simulink model "R_Mode_beta6"  (R2020a)
settings: Solver=FixedStepAuto  StartTime=0.0  StopTime=10.0  FixedStep=1e-3  RelTol=1e-3  EnableMultiTasking=on
undefined symbols (not defined in the file): D0, D1, D10, D11, D12, D13, D2, D3, D4, D5, D6, D7, D8, D9, PTA0, PTA1, PTA2, PTB23, PTB9, PTC16, PTC17, PTC2, PTC3, PTC4, PTD0, PTD1, PTD2, PTD3, square
libraries: frdmk64flib x20, simulink x2
settings Model: ExtModeTrigDuration=5  Creator=forre  LastModifiedBy=forre
settings OptimizationCC: EnhancedBackFolding=on  PassReuseOutputArgsAs=Individual arguments  ZeroExternalMemoryAtStartup=off  ZeroInternalMemoryAtStartup=off  MaxStackSize=64  OptimizeBlockOrder=speed  DifferentSizesBufferReuse=on  OptimizationCustomize=off  EfficientTunableParamExpr=on
settings DebuggingCC: ParameterTunabilityLossMsg=error
settings HardwareCC: ProdBitPerPointer=32  ProdBitPerSizeT=32  ProdBitPerPtrDiffT=32  ProdLargestAtomicInteger=Long  ProdLargestAtomicFloat=Double  ProdWordSize=32  ProdHWDeviceType=ARM Compatible->ARM Cortex
settings SFSimCC: MATLABDynamicMemAlloc=off
settings RTWCC: SystemTargetFile=ert.tlc  HardwareBoard=NXP FRDM-K64F  TemplateMakefile=ert_default_tmf  Toolchain=GNU Tools for ARM Embedded Processors
settings CodeAppCC: ForceParamTrailComments=on  IgnoreCustomStorageClasses=off  OperatorAnnotations=on  SimulinkDataObjDesc=on  SFDataObjDesc=on  InsertBlockDesc=on

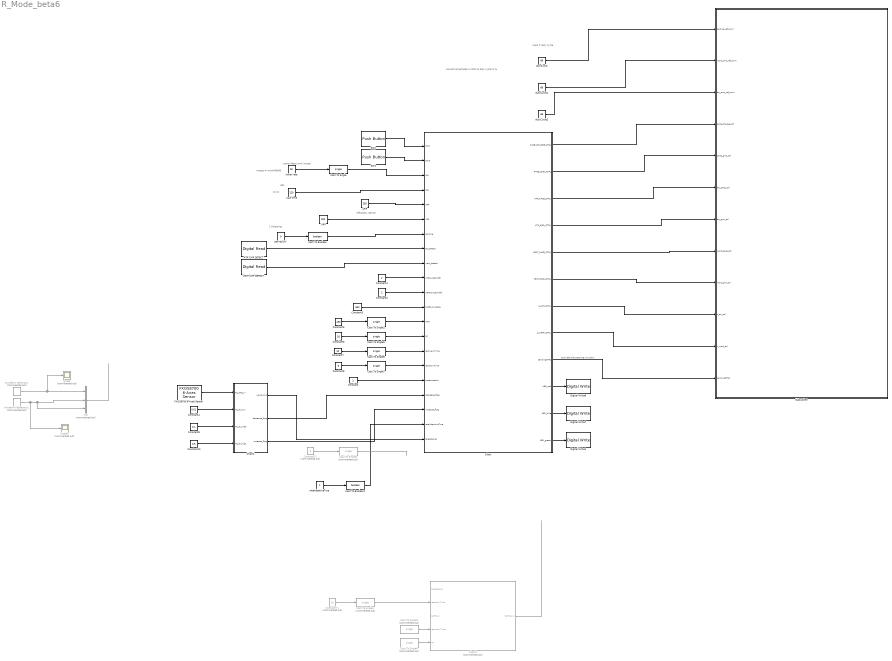
== system R_Mode_beta6 ==
  note: convert amplitude in Volts to duty cycle in %
  note: *****
  note: msecs = mins*60000
  note: URL
  note: refractory period
  note: Lower Rate Limit (msec)
  note: activate the sensing circuitry.
  note: input = duty cycle
  note: 1 if sensing
  ARP : Constant  Value=250
  ATR CMP DETECT : frdmk64flib/Digital Read  Whichpin=PTC16 (D0)  SampleTime=-1
  Cast To Boolean : DataTypeConversion  OutDataTypeStr=boolean
  Cast To Boolean1 : DataTypeConversion  OutDataTypeStr=boolean
  Cast To Single{,1,5..7} (5 alike) : DataTypeConversion  OutDataTypeStr=single
  Cast To Single{2..4,8} (4 alike) : DataTypeConversion  Commented=on  OutDataTypeStr=single
  Chart : Stateflow chart  TreatAsAtomicUnit=on
  Chart1 : Stateflow chart  TreatAsAtomicUnit=on
      settings: PortSchema="{\"entries\":[{\"content\":{\"sides\":[{\"content\":{\"connectorIds\":[\"In1\",\"In2\",\"In3\",\"In4\"]},\"type\":\"ConnectorPlacement.EquallySpacedRectSide\",\"uuid\":\"1efe160a-bf9a-41df-b710-bd83ffcce0b4\"},{\"content\":{\"connectorIds\":[\"Out1\",\"Out3\",\"Out2\"],\"side\":\"RIGHT\"},\"type\":\"ConnectorPlacement.EquallySpacedRectSide\",\"uuid\":\"ac30f416-04bb-4c91-9400-e1e71b20eb48\"},{\"content\":{\"connectorIds\":[],\"side\":\"TOP\"},\"type\":\"ConnectorPlacement.EquallySpacedRectSide\",\"uuid\":\"2c13bf7e-a139-4786-92e7-3ebc0a2be541\"}]},\"type\":\"ConnectorPlacement.EquallySpacedConnector\",\"uuid\":\"36ae9f3c-1d99-4fa5-b372-be33db95aa7c\"}],\"packageUris\":[\"http://schema.mathworks.com/mf0/Connector/19700101\"],\"version\":\"1.0\"}"
  Chart2 : Stateflow chart  Commented=on  TreatAsAtomicUnit=on
  Constant : Constant  Value=2  OutDataTypeStr=double
  Constant1 : Constant  Value=2
  Constant10 : Constant  Value=0.5  OutDataTypeStr=double
  Constant11 : Constant  Commented=on  Value=10  OutDataTypeStr=double
  Constant12 : Constant  Commented=on  Value=3  OutDataTypeStr=double
  Constant2 : Constant  Value=2
  Constant3 : Constant  Value=500
  Constant4 : Constant  Value=0.01  OutDataTypeStr=double
  Constant5 : Constant  Value=150  OutDataTypeStr=double
  Constant6 : Constant  Value=16  OutDataTypeStr=double
  Constant7 : Constant  Value=10  OutDataTypeStr=double
  Constant8 : Constant  Value=5  OutDataTypeStr=double
  Constant9 : Constant  Value=0.1  OutDataTypeStr=double
  Digital Write1 : frdmk64flib/Digital Write  Whichpin=GREEN_LED
  Digital Write6 : frdmk64flib/Digital Write  Whichpin=RED_LED
  Digital Write7 : frdmk64flib/Digital Write  Whichpin=BLUE_LED
  FXOS8700 6-Axes Sensor : frdmk64flib/FXOS8700 6-Axes Sensor  Activesensor=Accelerometer only  ODR=800Hz  HybridODR=400Hz  Accelfullrange=-2g to +2g  SampleTime=-1
  Mux : Mux  Commented=on  Inputs=3
  SW2 : frdmk64flib/Push Button  Whichswitch=SW2  SampleTime1=-1
  SW3 : frdmk64flib/Push Button  Whichswitch=SW3  SampleTime1=-1
  Scope : Scope  Commented=on
  Scope1 : Scope  Commented=on
  Subsystem : Subsystem
  VENT CMP DETECT : frdmk64flib/Digital Read  Whichpin=PTC17 (D1)  SampleTime=-1
  VRP : Constant  Value=250
  Waveform Generator : simulink/Sources/Waveform Generator  Commented=on  OutMin=[]  OutMax=[]  OutDataTypeStr=double  SelectedSignal=1  Signals=square(1,5,10,0)  BlockNames=MultiportSwitch_f97ce9ea1487498  SampleTime=0.1
  Waveform Generator1 : simulink/Sources/Waveform Generator  Commented=on  OutMin=[]  OutMax=[]  OutDataTypeStr=double  SelectedSignal=1  Signals=square(1,5,10,0)#  BlockNames=MultiportSwitch_5d833335861c4e9#MultiportSwitch_f0a91b941f4947f  SampleTime=0.1
  dutyCycle : Constant  Value=66
  dutyCycle1 : Constant  Value=66
  dutyCycle2 : Constant  Value=66
  lower rate : Constant  Value=50
  pacing ctrl : Constant  Value=0
  rateAdaptiveTrue : Constant
  wait time : Constant  Value=120
  wires:
  dutyCycle/1 -> Subsystem/1(pacing_ref_pwm)
  SW2/1 -> Chart/1(btn2)
  Chart/4(ATR_GND_CTRL) -> Subsystem/7(atr_gnd_ctrl)
  Constant1/1 -> Chart/10(ATRpulseWidth)
  Chart/3(ATR_PACE_CTRL) -> Subsystem/6(atr_pace_ctrl)
  Chart/1(PACE_CHARGE_CTRL) -> Subsystem/4(pace_charge_ctrl)
  Chart/2(PACE_GND_CTRL) -> Subsystem/5(pace_gnd_ctrl)
  lower rate/1 -> Cast To Single/1
  Chart/5(VENT_PACE_CTRL) -> Subsystem/8(vent_pace_ctrl)
  Chart/6(VENT_GND_CTRL) -> Subsystem/9(vent_gnd_ctrl)
  Chart/7(Z_ATR_CTRL) -> Subsystem/10(z_atr_ctrl)
  Chart/8(Z_VENT_CTRL) -> Subsystem/11(" z_vent_ctrl")
  pacing ctrl/1 -> Cast To Boolean/1
  ATR CMP DETECT/1 -> Chart/8(atr_detect)
  VENT CMP DETECT/1 -> Chart/9(vent_detect)
  dutyCycle1/1 -> Subsystem/2(vent_cmp_ref_pwm)
  dutyCycle2/1 -> Subsystem/3(atr_cmp_ref_pwm)
  Chart/9(sensingCTRL) -> Subsystem/12(sensingCTRL)
  Cast To Boolean/1 -> Chart/7(sensing)
  Chart/10(LED_red) -> Digital Write6/1
  Chart/11(LED_blue) -> Digital Write7/1
  SW3/1 -> Chart/2(btn3)
  wait time/1 -> Chart/4(URL)
  ARP/1 -> Chart/5(ARP)
  VRP/1 -> Chart/6(VRP)
  Constant2/1 -> Chart/11(VENTpulseWidth)
  Constant/1 -> Chart/17(paceLocation)
  Constant3/1 -> Chart/12(PACE_AV_delay)
  Chart1/1(Level_out) -> Chart/21(targetLevel)
  Constant5/1 -> Cast To Single1/1
  Constant4/1 -> Chart1/2(AC_th_low)
  Constant6/1 -> Cast To Single5/1
  Constant7/1 -> Cast To Single6/1
  Constant8/1 -> Cast To Single7/1
  Constant9/1 -> Chart1/3(AC_th_med)
  Constant10/1 -> Chart1/4(AC_th_high)
  FXOS8700 6-Axes Sensor/1 -> Chart1/1(AC_rate_in)
  Chart1/2(increase_flag) -> Chart/19(increase_flag)
  Chart1/3(decrease_flag) -> Chart/18(decrease_flag)
  Cast To Boolean1/1 -> Chart/20(rateAdaptiveTrue)
  rateAdaptiveTrue/1 -> Cast To Boolean1/1
  Chart2/1(RATE_out) -> ?
  ? -> Chart2/3(RATE_in)
  Constant11/1 -> Cast To Single2/1
  Cast To Single/1 -> Chart/3(LRL)
  Cast To Single1/1 -> Chart/13(MSR)
  Cast To Single2/1 -> Chart2/2(reactionTime)
  Cast To Single3/1 -> Chart2/4(recoveryTime)
  Cast To Single4/1 -> Chart2/5(RF)
  Cast To Single5/1 -> Chart/14(RF)
  Cast To Single6/1 -> Chart/15(recoveryTime)
  Cast To Single7/1 -> Chart/16(reactionTime)
  Chart/12(LED_green) -> Digital Write1/1
  Mux/1 -> ?
  Waveform Generator/1 -> Scope/1, Mux/1
  Waveform Generator1/1 -> Scope1/1, Mux/3, Mux/2
  Constant12/1 -> Cast To Single8/1
  Cast To Single8/1 -> ?

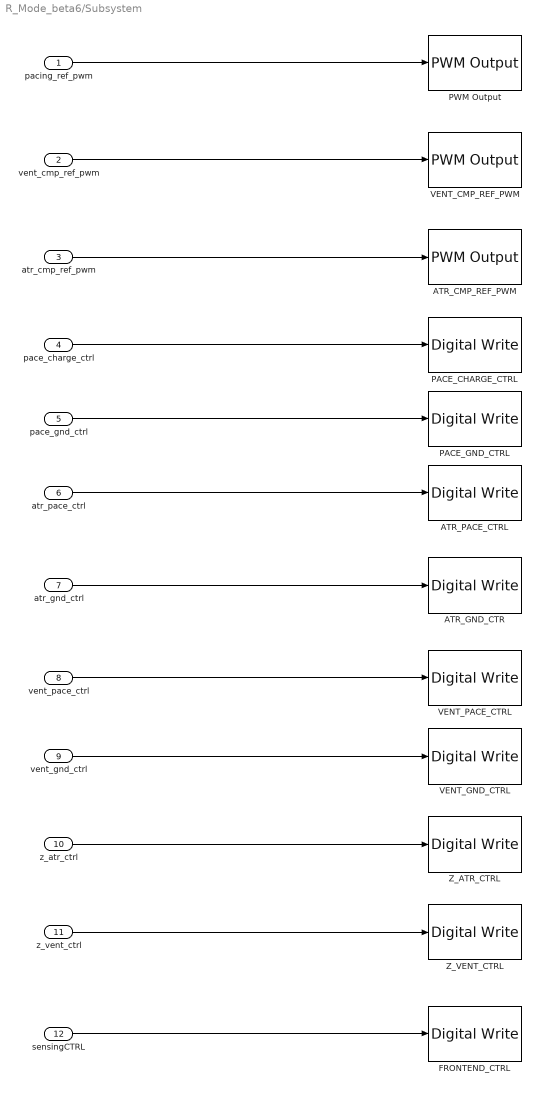
== system R_Mode_beta6/Subsystem ==
  pacing_ref_pwm : Inport
  vent_cmp_ref_pwm : Inport  Port=2
  atr_cmp_ref_pwm : Inport  Port=3
  pace_charge_ctrl : Inport  Port=4
  pace_gnd_ctrl : Inport  Port=5
  atr_pace_ctrl : Inport  Port=6
  atr_gnd_ctrl : Inport  Port=7
  vent_pace_ctrl : Inport  Port=8
  vent_gnd_ctrl : Inport  Port=9
  z_atr_ctrl : Inport  Port=10
  " z_vent_ctrl" : Inport  Port=11
  sensingCTRL : Inport  Port=12
  ATR_CMP_REF_PWM : frdmk64flib/PWM Output  Whichpin=PTC2 (D6)  InitialFrequency=2000  InitialDutyCycle=50
  ATR_GND_CTR : frdmk64flib/Digital Write  Whichpin=PTD2 (D11)
  ATR_PACE_CTRL : frdmk64flib/Digital Write  Whichpin=PTA0 (D8)
  FRONTEND_CTRL : frdmk64flib/Digital Write  Whichpin=PTD1 (D13)
  PACE_CHARGE_CTRL : frdmk64flib/Digital Write  Whichpin=PTB9 (D2)
  PACE_GND_CTRL : frdmk64flib/Digital Write  Whichpin=PTD0 (D10)
  PWM Output : frdmk64flib/PWM Output  Whichpin=PTA2 (D5)  InitialFrequency=2000  InitialDutyCycle=50
  VENT_CMP_REF_PWM : frdmk64flib/PWM Output  Whichpin=PTA1 (D3)  InitialFrequency=2000  InitialDutyCycle=50
  VENT_GND_CTRL : frdmk64flib/Digital Write  Whichpin=PTD3 (D12)
  VENT_PACE_CTRL : frdmk64flib/Digital Write  Whichpin=PTC4 (D9)
  Z_ATR_CTRL : frdmk64flib/Digital Write  Whichpin=PTB23 (D4)
  Z_VENT_CTRL : frdmk64flib/Digital Write  Whichpin=PTC3 (D7)
  wires:
  pace_gnd_ctrl/1 -> PACE_GND_CTRL/1
  atr_pace_ctrl/1 -> ATR_PACE_CTRL/1
  pace_charge_ctrl/1 -> PACE_CHARGE_CTRL/1
  atr_gnd_ctrl/1 -> ATR_GND_CTR/1
  vent_pace_ctrl/1 -> VENT_PACE_CTRL/1
  vent_gnd_ctrl/1 -> VENT_GND_CTRL/1
  z_atr_ctrl/1 -> Z_ATR_CTRL/1
  " z_vent_ctrl"/1 -> Z_VENT_CTRL/1
  sensingCTRL/1 -> FRONTEND_CTRL/1
  pacing_ref_pwm/1 -> PWM Output/1
  vent_cmp_ref_pwm/1 -> VENT_CMP_REF_PWM/1
  atr_cmp_ref_pwm/1 -> ATR_CMP_REF_PWM/1

== stateflow chart R_Mode_beta6/Chart ==
  note: if level = 0
      | RATE = LRL
      |
      | if level = 1
      | RATE = LRL + ResponseFactor
      |
      | if level = 2
      | RATE = LRL + 2*ResponseFactor
      |
      | if level = 3
      | RATE = LRL + 3*ResponseFactor
  note: IF target level > previous level
  note: target Level = LEVEL
  state INCREMENT_VENT [commented out]
    entry:
    incrementTime=reactionTime/((TargetLevel - PreviousLevel)*RF);
    % time/BPM increase
  note: incrementTime=reactionTime/((TargetLevel - PreviousLevel)*RF)
  note: R_MODE
  note: for VOO,VVI, so it don't go to REACTION_V and RECOVERY_V
  state adaptRATE_vent
    % RE factor need to time a rate (unit ppm)
    %it is depend on LRL and MSR values
    %RATE_out = RATE
    RATE = RATE + incrementAmount;
    LED_red = false;
    LED_blue= false;
    LED_green = false;
    %previousLevel = floor((RATE-LRL)/RF);
  state SENSING_VENT_TRUE
    entry:
    sensingCTRL = true;
  note: no change in RATE needed
  state VENT_CHARGING_AND_DISCHARGE
    entry:
    % for this state paceLocation = 1
    %begin charge and discharge cycle for ventricle
    msecPerPace = 60000.0/RATE; %new value in msec
    sensingCTRL = sensing; %enables the sensing circuitry if sensing = 1. Controled by input "sensing"
    ATR_PACE_CTRL = false;
    VENT_PACE_CTRL = false;
    PACE_CHARGE_CTRL = true;
    PACE_GND_CTRL = true;
    Z_VENT_CTRL = false;
    Z_ATR_CTRL = false
    VENT_GND_CTRL = true;
    ATR_GND_CTRL = false;
    LED_red = false;
  state VENT_PACING
    entry:
    % pace ventricle
    PACE_CHARGE_CTRL = false;
    PACE_GND_CTRL = true;
    VENT_PACE_CTRL = true;
    VENT_GND_CTRL = false;
    Z_VENT_CTRL = false;
    Z_ATR_CTRL = false;
    ATR_GND_CTRL = false;
    ATR_PACE_CTRL = false;
    sensingCTRL = sensing; %enables the sensing circuitry if sensing = 1. Controled by input "sensing"
    %VENT_P_flag = true; %pacing flag for V modes
    %recovery
    %recoveryTime_remaining = recoveryTime_remaining - (msecPerPace-VENTpulseWidth)
    LED_red=false;
  note: new Idea!
      |
      | secPerPace = msecPerPace/1000
      |
      | reactionTime/secPerPace = # of paces inside reactionTime
  note: INITIALIZE
  note: DECREMENT
  note: INCREMENT
  note: while targetLevel > previousLevel
  note: eg if reactionTIme = 10 and RATE = 60 BPM
      | 10/1 =10
      |
      | incrementAmount = (targetLevel-previousLevel)*RF/(# of paces inside reactionTime)
      |
      | so each cycle RATE = RATE + incrementAmount
  note: count = reactionTime/secPerPace = # of paces inside reactionTime
  note: beat sensed
  note: SWITCH TO VOO,VVI,VOOR,VVIR
  note: VENT PACING
  state RECOVERY_V [commented out]
    RATE = RATE - LEVEL*RE_factor
    % RE factor need to time a rate (unit ppm)
    %it is depend on LRL and MSR values
  state REACTION_V [commented out]
    RATE = RATE + LEVEL*RE_factor;
    % RE factor need to time a rate (unit ppm)
    %it is depend on LRL and MSR values
  note: SWITCH TO AOO, AAI,AOOR,AAIR
  state ATR_PACING [commented out]
    entry:
    % pace atrium
    PACE_GND_CTRL = true;
    VENT_PACE_CTRL = false;
    VENT_GND_CTRL = false;
    Z_VENT_CTRL = false;
    Z_ATR_CTRL = false;
    ATR_GND_CTRL = false;
    ATR_PACE_CTRL = true;
    sensingCTRL = sensing; %enables the sensing circuitry if sensing = 1. Controled by input "sensing"
    ATR_P_flag = true; %pacing flag for V modes
  note: SWITCH TO DOO,DOOR
  state ATR_CHARGING_AND_DISCHARGE [commented out]
    entry:
    % for this state paceLocation = 0
    %begin charge and discharge cycle for atrium
    msecPerPace = 60000/RATE; %new value for pace timing with msec units
    sensingCTRL = sensing; %enables the sensing circuitry if sensing = 1. Controled by input "sensing"
    ATR_PACE_CTRL = false;
    VENT_PACE_CTRL = false;
    PACE_CHARGE_CTRL = true;
    PACE_GND_CTRL = true;
    Z_VENT_CTRL = false;
    Z_ATR_CTRL = false;
    VENT_GND_CTRL = false;
    ATR_GND_CTRL = true;
  note: R_MODE
  note: ATR PACING
  note: SWITCH TO VOO,VVI,VOOR,VVIR
  state SENSING_ATR_TRUE [commented out]
    entry:
    sensingCTRL = true;
  note: beat sensed
  note: SWITCH TO DOO,DOOR
  state RECOVERY_V1 [commented out]
    RATE = RATE - LEVEL*RE_factor
    % RE factor need to time a rate (unit ppm)
    %it is depend on LRL and MSR values
  note: SWITCH TO AOO, AAI,AOOR,AAIR
  state REACTION_V1 [commented out]
    RATE = RATE + LEVEL*RE_factor;
    % RE factor need to time a rate (unit ppm)
    %it is depend on LRL and MSR values
  state DUAL_ATR_CHARGING_AND_DISCHARGE [commented out]
    entry:
    msecPerPace = 60000/RATE;
    % for this state paceLocation = 3
    %begin charge and discharge cycle for atrium
    ATR_PACE_CTRL = false;
    VENT_PACE_CTRL = false;
    PACE_CHARGE_CTRL = true;
    PACE_GND_CTRL = true;
    Z_VENT_CTRL = false;
    Z_ATR_CTRL = false;
    VENT_GND_CTRL = false;
    ATR_GND_CTRL = true;
  state DUAL_ATR_PACING [commented out]
    entry:
    % pace atrium
    PACE_GND_CTRL = true;
    VENT_PACE_CTRL = false;
    VENT_GND_CTRL = false;
    Z_VENT_CTRL = false;
    Z_ATR_CTRL = false;
    ATR_GND_CTRL = false;
    ATR_PACE_CTRL = true;
    AP_flag = true; % rise to true when Atrium have a pace
  note: DOO,DOOR
  state DUAL_VENT_PACING [commented out]
    entry:
    % pace ventricle
    PACE_GND_CTRL = true;
    VENT_PACE_CTRL = true;
    VENT_GND_CTRL = false;
    Z_VENT_CTRL = false;
    Z_ATR_CTRL = false;
    ATR_GND_CTRL = false;
    ATR_PACE_CTRL = false;
    sensingCTRL = sensing; %enables the sensing circuitry if sensing = 1. Controled by input "sensing"
    AP_flag = false;
  state DUAL_VENT_CHARGING_AND_DISCHARGE [commented out]
    entry:
    %begin charge and discharge cycle for ventricle
    msecPerPace = 60000/RATE; %new value in msec
    sensingCTRL = sensing; %enables the sensing circuitry if sensing = 1. Controled by input "sensing"
    ATR_PACE_CTRL = false;
    VENT_PACE_CTRL = false;
    PACE_CHARGE_CTRL = true;
    PACE_GND_CTRL = true;
    Z_VENT_CTRL = false;
    Z_ATR_CTRL = false
    VENT_GND_CTRL = true;
    ATR_GND_CTRL = false;
  INCREMENT_VENT -> INCREMENT_VENT [commented out] : after(incrementTime)[reactionTime_remaining>0]{RATE=RATE+1;reactionTime_remaining-incrementTime;}
  (junction 296) -> VENT_CHARGING_AND_DISCHARGE [order 1] : [rateAdaptiveTrue == false]
  INCREMENT_VENT -> INCREMENT_VENT [commented out] : [reactionTime_remaining <= 0]{previousLevel = LEVEL}
  VENT_PACING -> (junction 296) : after(VENTpulseWidth, msec)
  (junction 296) -> adaptRATE_vent [order 2] : [rateAdaptiveTrue == true]
  adaptRATE_vent -> adaptRATE_vent [order 3] : [increment_count <= 0 || decrement_count <=0]{previousLevel = targetLevel;LED_blue = true;LED_red = true;}
  adaptRATE_vent -> (junction 386) [order 2] : [targetLevel == previousLevel]{incrementAmount = 0;LED_green = true;}
  VENT_CHARGING_AND_DISCHARGE -> SENSING_VENT_TRUE [order 2] : after((VRP-VENTpulseWidth),msec)[sensing && (vent_detect || btn3)]
  SENSING_VENT_TRUE -> VENT_CHARGING_AND_DISCHARGE : after(VENTpulseWidth, msec)
  (junction 438) -> adaptRATE_vent [order 3]
  adaptRATE_vent -> (junction 438) [order 1] : [(incrementAmount ==0)&& ((targetLevel < previousLevel) || (targetLevel > previousLevel))]{increment_count = reactionTime*1000/msecPerPace;decrement_count = reactionTime*1000/msecPerPace;}
  adaptRATE_vent -> (junction 438) [order 4]
  (junction 438) -> (junction 386) [order 1] : [targetLevel < previousLevel]{incrementAmount = (targetLevel-previousLevel)*RF/(recoveryTime*1000/msecPerPace); decrement_count = decrement_count -1; LED_red = true;}
  (junction 438) -> (junction 386) [order 2] : [targetLevel > previousLevel]{incrementAmount = (targetLevel-previousLevel)*RF/(reactionTime*1000/msecPerPace); increment_count = increment_count -1; LED_blue = true;}
  (default) -> VENT_CHARGING_AND_DISCHARGE : {RATE = LRL;previousLevel = 0;incrementAmount=0;decrement_count = 0;increment_count = 0;}
  VENT_CHARGING_AND_DISCHARGE -> DUAL_ATR_CHARGING_AND_DISCHARGE [commented out] : [(paceLocation == 3) || (paceLocation == 6)]{RATE=LRL}
  (junction 386) -> VENT_CHARGING_AND_DISCHARGE [order 1] : [RATE< LRL]{RATE = LRL}
  (junction 386) -> VENT_CHARGING_AND_DISCHARGE [order 2] : [RATE>MSR]{RATE=MSR}
  (junction 386) -> VENT_CHARGING_AND_DISCHARGE [order 3]
  (junction 290) -> VENT_CHARGING_AND_DISCHARGE [commented out]
  DUAL_ATR_CHARGING_AND_DISCHARGE -> (junction 290) [commented out] : [(paceLocation == 2) || (paceLocation == 4)]{RATE=LRL}
  ATR_CHARGING_AND_DISCHARGE -> (junction 290) [commented out] : [(paceLocation == 2) || (paceLocation == 4)]{RATE=LRL}
  RECOVERY_V -> ? [commented out] : after(((RECOV_time/RE_factor)*60),sec){VENT_P_flag = false}
  VENT_CHARGING_AND_DISCHARGE -> VENT_PACING [order 1] : after((msecPerPace-VENTpulseWidth), msec)
  VENT_CHARGING_AND_DISCHARGE -> (junction 361) [commented out] : [(paceLocation==4)&&(VENT_P_flag== true)]
  (junction 361) -> VENT_CHARGING_AND_DISCHARGE [commented out] : [increase_flag == false]{VENT_P_flag = false}
  (junction 322) -> VENT_CHARGING_AND_DISCHARGE [commented out] : [(RATE>=MSR)]{RATE=MSR,VENT_P_flag = false}
  REACTION_V -> VENT_CHARGING_AND_DISCHARGE [commented out] : after((REACT_time/RE_factor),sec){VENT_P_flag = false}
  VENT_CHARGING_AND_DISCHARGE -> ATR_CHARGING_AND_DISCHARGE [commented out] : [(paceLocation == 1)|| (paceLocation == 5)]{RATE=LRL,ATR_P_flag = false}
  (junction 366) -> ? [commented out] : [(RATE<=LRL)]{RATE = LRL,VENT_P_flag = false}
  (default) -> (junction 326) [commented out] : [(paceLocation==4)&&(VENT_P_flag== true)]
  (junction 326) -> ? [commented out] : [decrease_flag == false]{VENT_P_flag = false}
  (junction 361) -> (junction 322) [commented out] : [increase_flag == true]
  (junction 326) -> (junction 366) [commented out] : [decrease_flag == true]
  (junction 366) -> RECOVERY_V [commented out] : [(RATE>LRL)]
  (junction 322) -> REACTION_V [commented out] : [RATE<MSR]
  (junction 347) -> ATR_CHARGING_AND_DISCHARGE [commented out] : [paceLocation == 1]{ATR_P_flag = false}
  ATR_PACING -> (junction 347) [commented out] : after(ATRpulseWidth, msec)
  (junction 347) -> ATR_CHARGING_AND_DISCHARGE [commented out] : [paceLocation == 5]
  ATR_CHARGING_AND_DISCHARGE -> (junction 282) [commented out] : [(paceLocation == 3) || (paceLocation == 6)]{RATE=LRL}
  ATR_CHARGING_AND_DISCHARGE -> (junction 353) [commented out] : [ATR_P_flag == false]
  (junction 353) -> ATR_PACING [commented out] : after((msecPerPace-ATRpulseWidth), msec){PACE_CHARGE_CTRL = false;}
  RECOVERY_V1 -> ATR_CHARGING_AND_DISCHARGE [commented out] : after(((RECOV_time/RE_factor)*60),sec){ATR_P_flag = false}
  REACTION_V1 -> ATR_CHARGING_AND_DISCHARGE [commented out] : after((REACT_time/RE_factor),sec){ATR_P_flag = false}
  (junction 341) -> ATR_CHARGING_AND_DISCHARGE [commented out] : [RATE<=LRL]{RATE = LRL,ATR_P_flag = false}
  (junction 331) -> ATR_CHARGING_AND_DISCHARGE [commented out] : [LEVEL==0]{RATE = LRL,ATR_P_flag = false}
  ATR_CHARGING_AND_DISCHARGE -> (junction 341) [commented out] : [(paceLocation==5)&&(ATR_P_flag== true)]
  ATR_CHARGING_AND_DISCHARGE -> SENSING_ATR_TRUE [commented out] : after((ARP-ATRpulseWidth),msec)[sensing && (atr_detect || btn3)]
  SENSING_ATR_TRUE -> ATR_CHARGING_AND_DISCHARGE [commented out] : after(ATRpulseWidth, msec)
  DUAL_ATR_CHARGING_AND_DISCHARGE -> ATR_CHARGING_AND_DISCHARGE [commented out] : [(paceLocation == 1)|| (paceLocation == 5)]{RATE=LRL,ATR_P_flag == false}
  ATR_CHARGING_AND_DISCHARGE -> (junction 336) [commented out] : [(paceLocation==5)&&(ATR_P_flag== true)]
  (junction 336) -> ATR_CHARGING_AND_DISCHARGE [commented out] : [RATE>=MSR]{RATE=MSR,ATR_P_flag = false}
  (junction 341) -> RECOVERY_V1 [commented out] : [RATE>LRL]
  (junction 336) -> (junction 331) [commented out] : [RATE<MSR]
  (junction 331) -> REACTION_V1 [commented out] : [LEVEL>0]
  (junction 282) -> DUAL_ATR_CHARGING_AND_DISCHARGE [commented out] : {AP_flag == false}
  DUAL_ATR_CHARGING_AND_DISCHARGE -> DUAL_ATR_PACING [commented out] : [AP_flag == false]{PACE_CHARGE_CTRL = false;}
  DUAL_ATR_PACING -> DUAL_ATR_CHARGING_AND_DISCHARGE [commented out] : after( ATRpulseWidth, msec)
  DUAL_ATR_CHARGING_AND_DISCHARGE -> (junction 285) [commented out] : [AP_flag == true]
  (junction 285) -> DUAL_VENT_CHARGING_AND_DISCHARGE [commented out] : after(PACE_AV_delay-ATRpulseWidth,msec)
  (junction 288) -> DUAL_ATR_CHARGING_AND_DISCHARGE [commented out] : [AP_flag == false]
  DUAL_VENT_PACING -> DUAL_VENT_CHARGING_AND_DISCHARGE [commented out] : after((VENTpulseWidth), msec)
  DUAL_VENT_CHARGING_AND_DISCHARGE -> DUAL_VENT_PACING [commented out] : [AP_flag == true]{PACE_CHARGE_CTRL = false;}
  DUAL_VENT_CHARGING_AND_DISCHARGE -> (junction 288) [commented out] : after(msecPerPace-VENTpulseWidth-PACE_AV_delay,msec)
  data: PACE_CHARGE_CTRL output boolean; PACE_GND_CTRL output boolean; btn2 input boolean; btn3 input boolean; ATR_PACE_CTRL output boolean; ATR_GND_CTRL output boolean; LRL input single; URL input double; ARP input double; VRP input double; VENT_PACE_CTRL output boolean; VENT_GND_CTRL output boolean; Z_ATR_CTRL output boolean; Z_VENT_CTRL output boolean; sensing input boolean; atr_detect input boolean; vent_detect input boolean; sensingCTRL output boolean; msecPerPace local single; ATRpulseWidth input double; VENTpulseWidth input double; PACE_AV_delay input double; AP_flag local boolean; MSR input single; RF input single; recoveryTime input single; reactionTime input single; paceLocation input double; ATR_P_flag local boolean; VENT_P_flag local boolean; RATE local single; decrease_flag input boolean; increase_flag input boolean; rateAdaptiveTrue input boolean; LED_red output boolean; targetLevel input single; previousLevel local single; decrement_count local single; incrementAmount local single; increment_count local single; LED_blue output boolean; LED_green output boolean
  data atr_detect settings: description=|
      | 0 = pace atrium
      | 1 = pace ventricle
  data vent_detect settings: description=|
      | 0 = pace atrium
      | 1 = pace ventricle
  data paceLocation settings: description=|
      | 0 = pace atrium
      | 1 = pace ventricle

== stateflow chart R_Mode_beta6/Chart2 ==
  note: if level = 0
      | RATE = LRL
      |
      | if level = 1
      | RATE = LRL + ResponseFactor
      |
      | if level = 2
      | RATE = LRL + 2*ResponseFactor
      |
      | if level = 3
      | RATE = LRL + 3*ResponseFactor
  state START
    entry:
    reactionTime_remaining = reactionTime;
    recoveryTime_remaining = recoveryTime;
    RATE_out = RATE_in;
  note: incrementTime=reactionTime/((TargetLevel - PreviousLevel)*RF)
  note: IF target level > previous level
  note: IF target level < previous level
  note: decrease
  note: Increase
  state INCREMENT
    entry:
    incrementTime=reactionTime/((targetLevel - previousLevel)*RF);
    % time/BPM increase
  state DECREMENT
    entry:
    decrementTime=recoveryTime/((previousLevel - targetLevel)*RF);
    % time/BPM increase
  (default) -> START : {previousLevel = 0;}
  START -> INCREMENT [order 1] : [targetLevel > previousLevel]
  INCREMENT -> START [order 1] : [targetLevel <= previousLevel]
  DECREMENT -> START [order 1] : [targetLevel >= previousLevel]
  START -> DECREMENT [order 2] : [targetLevel < previousLevel]
  DECREMENT -> DECREMENT [order 3] : after(decrementTime, sec)[recoveryTime_remaining>0]{RATE_out=RATE_in+1;recoveryTime_remaining-decrementTime;}
  INCREMENT -> INCREMENT [order 3] : after(incrementTime,sec)[reactionTime_remaining>0]{RATE_out=RATE_in+1;reactionTime_remaining-incrementTime;}
  DECREMENT -> DECREMENT [order 2] : [recoveryTime_remaining <= 0]{previousLevel = targetLevel}
  INCREMENT -> INCREMENT [order 2] : [reactionTime_remaining <= 0]{previousLevel = targetLevel}
  data: targetLevel input single; reactionTime input single; RATE_out output single; RATE_in input single; previousLevel local single; recoveryTime input single; decrementTime local single; incrementTime local single; reactionTime_remaining local; recoveryTime_remaining local; RF input single

== stateflow chart R_Mode_beta6/Chart1 ==
  note: any of the directions > HIGH (running)
  note: ALL Directions <= LOW (still)
  state rest
    Level_out = 0;
    prev_level = 0;
  state Get_data
    AC_x = abs(AC_rate_in(1));
    AC_y = abs(AC_rate_in(2));
    AC_z = abs(AC_rate_in(3));
  state high
    Level_out = 3;
    prev_level = 3;
  note: any direction <= MED (walking)
  state low
    Level_out = 1;
    prev_level = 1;
  state med
    Level_out = 2;
    prev_level = 2;
  (junction 72) -> Get_data [order 2] : [prev_level==3]{increase_flag = false;decrease_flag = false;}
  (default) -> Get_data
  Get_data -> rest [order 1] : [AC_x<= AC_th_low && AC_y<=AC_th_low && AC_z <=AC_th_low]{decrease_flag = false;increase_flag = false;}
  rest -> Get_data
  Get_data -> (junction 72) [order 4] : [AC_x>= AC_th_high || AC_y>= AC_th_high  || AC_z >= AC_th_high]
  (junction 72) -> high [order 1] : [prev_level<3]{increase_flag = true;decrease_flag = false;}
  high -> Get_data
  Get_data -> (junction 67) [order 2] : [AC_x<= AC_th_med || AC_y<= AC_th_med  || AC_z <= AC_th_med]
  Get_data -> (junction 60) [order 3] : [AC_x<= AC_th_high || AC_y<= AC_th_high  || AC_z <= AC_th_high]
  low -> Get_data
  med -> Get_data
  (junction 60) -> med [order 1] : [prev_level<2]{increase_flag = true;decrease_flag = false;}
  (junction 60) -> med [order 2] : [prev_level >2]{decrease_flag = true;increase_flag = false;}
  (junction 60) -> med [order 3] : [prev_level==2]{increase_flag = false;decrease_flag = false;}
  (junction 67) -> low [order 1] : [prev_level >1]{decrease_flag = true;increase_flag = false;}
  (junction 67) -> low [order 2] : [prev_level<1]{increase_flag = true;decrease_flag = false;}
  (junction 67) -> low [order 3] : [prev_level==1]{increase_flag = false;decrease_flag = false;}
  data: AC_rate_in input; Level_out output single; AC_th_low input; AC_th_med input; AC_th_high input; AC_x local; AC_y local; AC_z local; AC_th_x local; AC_th_y local; AC_th_z local; increase_flag output boolean; prev_level local double; decrease_flag output boolean
